simulink model "TopDE3340Board"  (Simulink 7.6)
settings: Solver=ode45  StartTime=0.0  StopTime=10.0  RelTol=1e-3
InitFcn:
  | %% DSPBuilder Start
  | alt_dspbuilder_update_model(bdroot)
  | %% DSPBuilder End
libraries: allblocks_alteradspbuilder2 x36, Stratix_III_DE3_340_alteradspbuilder2 x1
settings Model: Creator=lkong  LastModifiedBy=akarapet
settings DataIOCC: SignalLoggingName=sigsOut
settings OptimizationCC: InlineInvariantSignals=on  InitFltsAndDblsToZero=on
settings DebuggingCC: SaveWithParameterizedLinksMsg=none  SignalResolutionControl=TryResolveAllWithWarning  SolverPrmCheckMsg=none  MultiTaskDSMMsg=warning  MultiTaskCondExecSysMsg=none  StrictBusMsg=Warning
settings HardwareCC: TargetUnknown=on
settings RTWCC: IncludeERTFirstTime=on
settings GRTTargetCC: TargetFcnLib=ansi_tfl_tmw.mat

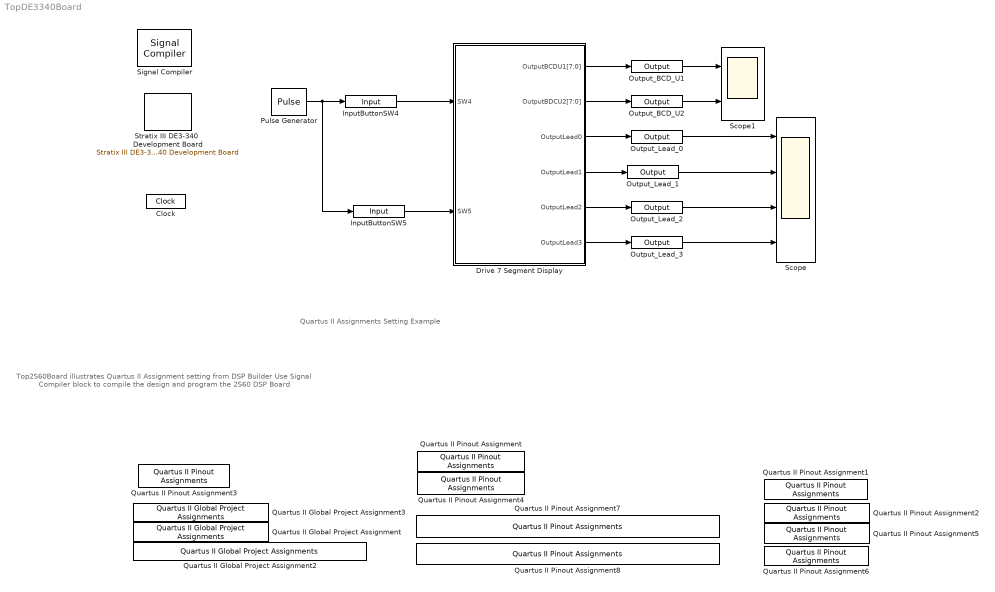
== system TopDE3340Board ==
  note: Quartus II Assignments Setting Example
  note: Top2S60Board illustrates Quartus II Assignment setting from DSP Builder
      |
      | Use Signal Compiler block to compile the design and program the 2S60 DSP Board
  Clock : allblocks_alteradspbuilder2/Clock  ClockPeriod=100  ClockPeriodUnit=ns  SampleTime=1  ResetLatency=0  ResetRegisterCascadeDepth=0  SimulationStartCycle=5  PhaseOffset=0  Reset=aclr  ResetType=Active Low  Export=off
  Drive 7 Segment Display : Subsystem  AncestorBlock=ALTELINK/AltLab/HDL SubSystem
      mask Type: SubSystem AlteraBlockSet
  InputButtonSW4 : allblocks_alteradspbuilder2/Input  iofile=/data/akarapet/qshell_linux64_test/p4/dsp_builder/dsp_builder2/Documentation/DesignExamples/Demos/QuartusIIConstraints/tb_TopDE3340Board/TopDE3340Board_InputButtonSW4.salt  BusType=Single Bit  bwl=1  bwr=0  SpecifyClock=off  PORTTYPE=Input  externalType=Inferred  allowFloatingPointOverride=on  logOutputs=off
  InputButtonSW5 : allblocks_alteradspbuilder2/Input  iofile=/data/akarapet/qshell_linux64_test/p4/dsp_builder/dsp_builder2/Documentation/DesignExamples/Demos/QuartusIIConstraints/tb_TopDE3340Board/TopDE3340Board_InputButtonSW5.salt  BusType=Single Bit  bwl=1  bwr=0  SpecifyClock=off  PORTTYPE=Input  externalType=Inferred  allowFloatingPointOverride=on  logOutputs=off
  Output_BCD_U1 : allblocks_alteradspbuilder2/Output  iofile=/data/akarapet/qshell_linux64_test/p4/dsp_builder/dsp_builder2/Documentation/DesignExamples/Demos/QuartusIIConstraints/tb_TopDE3340Board/TopDE3340Board_Output%5FBCD%5FU1.capture  BusType=Unsigned Integer  bwl=8  bwr=0  externalType=Inferred  PORTTYPE=Output  allowFloatingPointOverride=on  logOutputs=off
  Output_BCD_U2 : allblocks_alteradspbuilder2/Output  iofile=/data/akarapet/qshell_linux64_test/p4/dsp_builder/dsp_builder2/Documentation/DesignExamples/Demos/QuartusIIConstraints/tb_TopDE3340Board/TopDE3340Board_Output%5FBCD%5FU2.capture  BusType=Unsigned Integer  bwl=8  bwr=0  externalType=Inferred  PORTTYPE=Output  allowFloatingPointOverride=on  logOutputs=off
  Output_Lead_0 : allblocks_alteradspbuilder2/Output  iofile=/data/akarapet/qshell_linux64_test/p4/dsp_builder/dsp_builder2/Documentation/DesignExamples/Demos/QuartusIIConstraints/tb_TopDE3340Board/TopDE3340Board_Output%5FLead%5F0.capture  BusType=Single Bit  bwl=1  bwr=0  externalType=Inferred  PORTTYPE=Output  allowFloatingPointOverride=on  logOutputs=off
  Output_Lead_1 : allblocks_alteradspbuilder2/Output  iofile=/data/akarapet/qshell_linux64_test/p4/dsp_builder/dsp_builder2/Documentation/DesignExamples/Demos/QuartusIIConstraints/tb_TopDE3340Board/TopDE3340Board_Output%5FLead%5F1.capture  BusType=Single Bit  bwl=1  bwr=0  externalType=Inferred  PORTTYPE=Output  allowFloatingPointOverride=on  logOutputs=off
  Output_Lead_2 : allblocks_alteradspbuilder2/Output  iofile=/data/akarapet/qshell_linux64_test/p4/dsp_builder/dsp_builder2/Documentation/DesignExamples/Demos/QuartusIIConstraints/tb_TopDE3340Board/TopDE3340Board_Output%5FLead%5F2.capture  BusType=Single Bit  bwl=1  bwr=0  externalType=Inferred  PORTTYPE=Output  allowFloatingPointOverride=on  logOutputs=off
  Output_Lead_3 : allblocks_alteradspbuilder2/Output  iofile=/data/akarapet/qshell_linux64_test/p4/dsp_builder/dsp_builder2/Documentation/DesignExamples/Demos/QuartusIIConstraints/tb_TopDE3340Board/TopDE3340Board_Output%5FLead%5F3.capture  BusType=Single Bit  bwl=1  bwr=0  externalType=Inferred  PORTTYPE=Output  allowFloatingPointOverride=on  logOutputs=off
  Pulse Generator : DiscretePulseGenerator  Period=20000  PulseWidth=2
  Quartus II Global Project Assignment : allblocks_alteradspbuilder2/Quartus II Global Project Assignments  QuartusIIAssignmentName=TCO_REQUIREMENT  QuartusIIAssignmentValue=10ns
  Quartus II Global Project Assignment2 : allblocks_alteradspbuilder2/Quartus II Global Project Assignments  QuartusIIAssignmentName=RESERVE_ALL_UNUSED_PINS  QuartusIIAssignmentValue="\"AS INPUT TRI-STATED\""
  Quartus II Global Project Assignment3 : allblocks_alteradspbuilder2/Quartus II Global Project Assignments  QuartusIIAssignmentName=TSU_REQUIREMENT  QuartusIIAssignmentValue=10ns
  Quartus II Pinout Assignment : allblocks_alteradspbuilder2/Quartus II Pinout Assignments  QuartusIIAssignmentName=InputButtonSW4  QuartusIIAssignmentValue=Pin_W5
  Quartus II Pinout Assignment1 : allblocks_alteradspbuilder2/Quartus II Pinout Assignments  QuartusIIAssignmentName=Output_Lead_0  QuartusIIAssignmentValue=Pin_AD1
  Quartus II Pinout Assignment2 : allblocks_alteradspbuilder2/Quartus II Pinout Assignments  QuartusIIAssignmentName=Output_Lead_1  QuartusIIAssignmentValue=Pin_AC1
  Quartus II Pinout Assignment3 : allblocks_alteradspbuilder2/Quartus II Pinout Assignments  QuartusIIAssignmentName=clock  QuartusIIAssignmentValue=Pin_T33
  Quartus II Pinout Assignment4 : allblocks_alteradspbuilder2/Quartus II Pinout Assignments  QuartusIIAssignmentName=InputButtonSW5  QuartusIIAssignmentValue=Pin_W6
  Quartus II Pinout Assignment5 : allblocks_alteradspbuilder2/Quartus II Pinout Assignments  QuartusIIAssignmentName=Output_Lead_2  QuartusIIAssignmentValue=Pin_AC2
  Quartus II Pinout Assignment6 : allblocks_alteradspbuilder2/Quartus II Pinout Assignments  QuartusIIAssignmentName=Output_Lead_3  QuartusIIAssignmentValue=Pin_AB2
  Quartus II Pinout Assignment7 : allblocks_alteradspbuilder2/Quartus II Pinout Assignments  QuartusIIAssignmentName=Output_BCD_U1  QuartusIIAssignmentValue=Pin_V3, Pin_W12, Pin_Y11, Pin_W10, Pin_W8, Pin_W7, Pin_Y5, Pin_Y6
  Quartus II Pinout Assignment8 : allblocks_alteradspbuilder2/Quartus II Pinout Assignments  QuartusIIAssignmentName=Output_BCD_U2  QuartusIIAssignmentValue=Pin_V4, Pin_P3, Pin_N4, Pin_N3, Pin_N1, Pin_M1, Pin_L1, Pin_L2
  Scope : Scope  NumInputPorts=4
      settings: YMin=-5~-5~-5~-5  YMax=5~5~5~5
  Scope1 : Scope  NumInputPorts=2
      settings: YMin=-5~-5  YMax=5~5
  Signal Compiler : allblocks_alteradspbuilder2/Signal Compiler  DeviceFamily=Stratix III  DeviceName=EP3SL340F1152C3  EnableSignalTap=off  SignalTapDepth=128  UseBoardBlock=on  StpUseDefaultClock=on  StpClock=Clock  ExportDir=/home/akarapet
  Stratix III DE3-340  Development Board : Stratix_III_DE3_340_alteradspbuilder2/Stratix III DE3-340 Development Board  ClockPinIn=Pin_T33  GlobalResetPin=Pin_U31  device=EP3SL340F1152C3
  wires:
  InputButtonSW4/1 -> Drive 7 Segment Display/1(SW4)
  InputButtonSW5/1 -> Drive 7 Segment Display/2(SW5)
  Drive 7 Segment Display/1(OutputBCDU1[7:0]) -> Output_BCD_U1/1
  Drive 7 Segment Display/2(OutputBDCU2[7:0]) -> Output_BCD_U2/1
  Output_Lead_0/1 -> Scope/1
  Output_Lead_1/1 -> Scope/2
  Output_Lead_2/1 -> Scope/3
  Output_Lead_3/1 -> Scope/4
  Pulse Generator/1 -> InputButtonSW4/1, InputButtonSW5/1
  Output_BCD_U1/1 -> Scope1/1
  Drive 7 Segment Display/3(OutputLead0) -> Output_Lead_0/1
  Drive 7 Segment Display/4(OutputLead1) -> Output_Lead_1/1
  Drive 7 Segment Display/5(OutputLead2) -> Output_Lead_2/1
  Drive 7 Segment Display/6(OutputLead3) -> Output_Lead_3/1
  Output_BCD_U2/1 -> Scope1/2

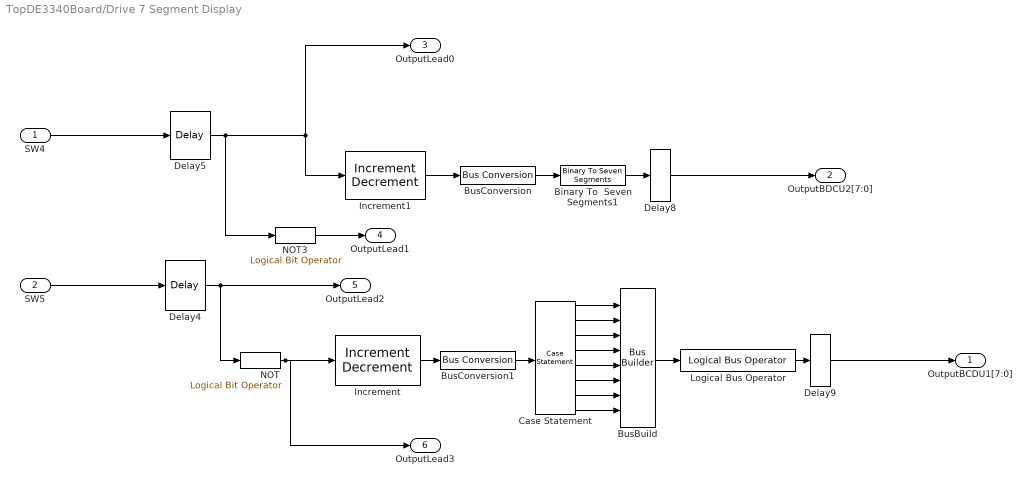
== system TopDE3340Board/Drive 7 Segment Display ==
  SW4 : Inport
  SW5 : Inport  Port=2
  Binary To  Seven Segments1 : allblocks_alteradspbuilder2/Binary To Seven Segments  pipeline_display=0
  BusBuild : allblocks_alteradspbuilder2/Bus Builder  BusType=Unsigned Integer  bwl=8  bwr=0  pipeline_display=0
  BusConversion : allblocks_alteradspbuilder2/Bus Conversion  BusType=Unsigned Integer  ibwl=31  ibwr=0  bwl=4  bwr=0  bitToConnectToOutputLSB=25  round=off  saturate=off  pipeline_display=0
  BusConversion1 : allblocks_alteradspbuilder2/Bus Conversion  BusType=Unsigned Integer  ibwl=26  ibwr=0  bwl=3  bwr=0  bitToConnectToOutputLSB=23  round=off  saturate=off  pipeline_display=0
  Case Statement : allblocks_alteradspbuilder2/Case Statement  numOutputs=8  case_expression=0,1,2,3,4,5,6  formatted_case_expression=00000000,00000001,00000010,00000011,00000100,00000101,00000110  BusType=Signed Integer  bwl=8  bwr=0  pipeline=on  pipeline_display=1  hasDefault=on
  Delay4 : allblocks_alteradspbuilder2/Delay  pipeline=1  pipeline_display=1  ClockPhase=1  use_ena=off  use_sclr=off  allowFloatingPointOverride=on  logOutputs=off  logFile=/data/akarapet/qshell_linux64_test/p4/dsp_builder/dsp_builder2/Documentation/DesignExamples/Demos/QuartusIIConstraints/tb_TopDE3340Board/TopDE3340Board_Drive+7+Segment+Display_Delay4.fixedpointlog  use_init=off  reset_value=1
  Delay5 : allblocks_alteradspbuilder2/Delay  pipeline=1  pipeline_display=1  ClockPhase=1  use_ena=off  use_sclr=off  allowFloatingPointOverride=on  logOutputs=off  logFile=/data/akarapet/qshell_linux64_test/p4/dsp_builder/dsp_builder2/Documentation/DesignExamples/Demos/QuartusIIConstraints/tb_TopDE3340Board/TopDE3340Board_Drive+7+Segment+Display_Delay5.fixedpointlog  use_init=off  reset_value=1
  Delay8 : allblocks_alteradspbuilder2/Delay  pipeline=1  pipeline_display=1  ClockPhase=1  use_ena=off  use_sclr=off  allowFloatingPointOverride=on  logOutputs=off  logFile=/data/akarapet/qshell_linux64_test/p4/dsp_builder/dsp_builder2/Documentation/DesignExamples/Demos/QuartusIIConstraints/tb_TopDE3340Board/TopDE3340Board_Drive+7+Segment+Display_Delay8.fixedpointlog  use_init=off  reset_value=1
  Delay9 : allblocks_alteradspbuilder2/Delay  pipeline=1  pipeline_display=1  ClockPhase=1  use_ena=off  use_sclr=off  allowFloatingPointOverride=on  logOutputs=off  logFile=/data/akarapet/qshell_linux64_test/p4/dsp_builder/dsp_builder2/Documentation/DesignExamples/Demos/QuartusIIConstraints/tb_TopDE3340Board/TopDE3340Board_Drive+7+Segment+Display_Delay9.fixedpointlog  use_init=off  reset_value=1
  Increment : allblocks_alteradspbuilder2/Increment Decrement  BusType=Unsigned Integer  bwl=26  bwr=0  SpecifyClock=off  clr_value=0  direction=Increment  phase_selection=1  use_ena=on  use_sclr=off  pipeline_display=1
  Increment1 : allblocks_alteradspbuilder2/Increment Decrement  BusType=Unsigned Integer  bwl=29  bwr=0  SpecifyClock=off  clr_value=0  direction=Increment  phase_selection=1  use_ena=on  use_sclr=off  pipeline_display=1
  Logical Bus Operator : allblocks_alteradspbuilder2/Logical Bus Operator  BusType=Signed Fractional  bwl=8  bwr=0  LogicalOp_text=Invert  mask_value_num=-5  shift_amount=3  force_sign_ext=off  pipeline_display=0
  NOT : allblocks_alteradspbuilder2/Logical Bit Operator  LogicalOperator=NOT  user_inputs=2  pipeline_display=0
  NOT3 : allblocks_alteradspbuilder2/Logical Bit Operator  LogicalOperator=NOT  user_inputs=2  pipeline_display=0
  OutputBCDU1[7:0] : Outport
  OutputBDCU2[7:0] : Outport  Port=2
  OutputLead0 : Outport  Port=3
  OutputLead1 : Outport  Port=4
  OutputLead2 : Outport  Port=5
  OutputLead3 : Outport  Port=6
  wires:
  Increment1/1 -> BusConversion/1
  BusConversion/1 -> Binary To  Seven Segments1/1
  Increment/1 -> BusConversion1/1
  Delay4/1 -> NOT/1, OutputLead2/1
  Delay5/1 -> NOT3/1, Increment1/1, OutputLead0/1
  NOT/1 -> Increment/1, OutputLead3/1
  NOT3/1 -> OutputLead1/1
  Binary To  Seven Segments1/1 -> Delay8/1
  Case Statement/8 -> BusBuild/8
  Case Statement/1 -> BusBuild/1
  Case Statement/2 -> BusBuild/2
  Case Statement/3 -> BusBuild/3
  Case Statement/4 -> BusBuild/4
  Case Statement/5 -> BusBuild/5
  Case Statement/6 -> BusBuild/6
  Case Statement/7 -> BusBuild/7
  BusBuild/1 -> Logical Bus Operator/1
  BusConversion1/1 -> Case Statement/1
  Logical Bus Operator/1 -> Delay9/1
  Delay8/1 -> OutputBDCU2[7:0]/1
  Delay9/1 -> OutputBCDU1[7:0]/1
  SW4/1 -> Delay5/1
  SW5/1 -> Delay4/1
